simulink model "outputpwa"  (Simulink 5.0)
settings: Solver=ode45  StartTime=0.0  StopTime=Tstop  RelTol=1e-3
values from neighbouring files (symbols this model uses):
  C = hybcon(S,Q,N,limits,refs)    [binary_inputs_sim.m]    (also in bm99benchmark.m; bm99norm2.m; bm99sim.m; exp2mld_mimo.m = lincon(model,'track',cost,interval,limits))
  P = pwa(S)    [bball.m]    (also in bm99sim.m; heatcool.m; logicstatesim.m; supply_chain.m)
libraries: hyblib x2
settings Model: LastModifiedBy=Alberto Bemporad

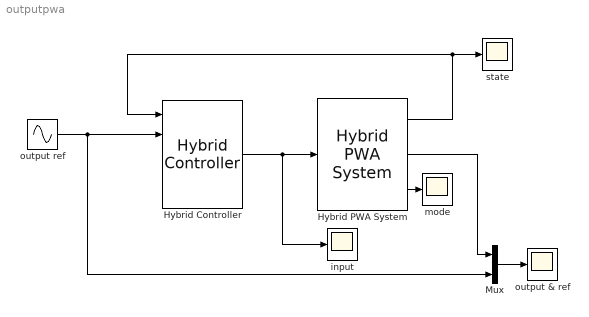
== system outputpwa ==
  Hybrid Controller : hyblib/Hybrid Controller  C=C  S=S
  Hybrid PWA System : hyblib/Hybrid PWA System  P=P  x0init=x0
  Mux : Mux  Inputs=2
  input : Scope
      settings: TimeRange=100  YMin=-1  YMax=0.4  SaveName=ScopeData2
  mode : Scope
  output & ref : Scope
      settings: TimeRange=100  YMin=-1  YMax=1  SaveName=ScopeData4
  output ref : Sin  Frequency=1/8  SampleTime=0
  state : Scope
      settings: SaveName=ScopeData3
  wires:
  Hybrid Controller/1 -> input/1, Hybrid PWA System/1
  Hybrid PWA System/1 -> state/1, Hybrid Controller/1
  output ref/1 -> Hybrid Controller/2, Mux/2
  Mux/1 -> output & ref/1
  Hybrid PWA System/3 -> mode/1
  Hybrid PWA System/2 -> Mux/1
